simulink model "gyroscope"  (R2018a)
settings: Solver=VariableStepAuto  StartTime=0.0  StopTime=10.0  RelTol=1e-3
libraries: simulink_extras x3
settings Model: Creator=David  LastModifiedBy=David

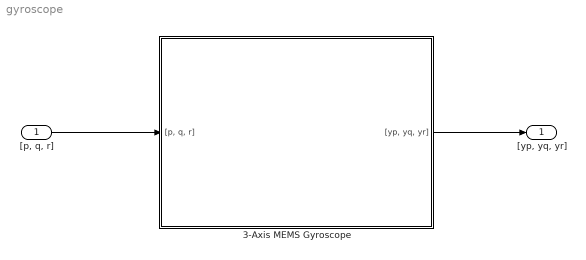
== system gyroscope ==
  "[p, q, r]" : Inport
  3-Axis MEMS Gyroscope : Subsystem  mask{SampleTime=0.01, gyroXNoiseDensity=0, gyroYNoiseDensity=0, gyroZNoiseDensity=0, gyroXBandwidthHz=1E06, gyroYBandwidthHz=1E06, gyroZBandwidthHz=1E06, gyroXInit=0, gyroYInit=0, gyroZInit=0, gyroXUpperSaturation=inf, gyroXLowerSaturation=-inf, gyroYUpperSaturation=inf, gyroYLowerSaturation=-inf, gyroZUpperSaturation=inf, gyroZLowerSaturation=-inf, gyroXResolution=1E-06, gyroYResolution=1E-06, gyroZResolution=1E-06}
      mask prompts: SampleTime "Gyroscope Sample Time (s)"; gyroXNoiseDensity "X Gyroscope Noise Density (rad/s/sqrt(Hz))"; gyroYNoiseDensity "Y Gyroscope Noise Density (rad/s/sqrt(Hz))"; gyroZNoiseDensity "Z Gyroscope Noise Density (rad/s/sqrt(Hz))"; gyroXBandwidthHz "X Gyroscope Bandwidth (Hz)"; gyroYBandwidthHz "Y Gyroscope Bandwidth (Hz)"; gyroZBandwidthHz "Z Gyroscope Bandwidth (Hz)"; gyroXInit "X Gyroscope Initial Condition (rad/s)"; gyroYInit "Y Gyroscope Initial Condition (rad/s)"; gyroZInit "Z Gyroscope Initial Condition (rad/s)"; gyroXUpperSaturation "X Gyroscope Measurement Upper Saturation Limit (rad/s)"; gyroXLowerSaturation "X Gyroscope Measurement Lower Saturation Limit (rad/s)"; gyroYUpperSaturation "Y Gyroscope Measurement Upper Saturation Limit (rad/s)"; gyroYLowerSaturation "Y Gyroscope Measurement Lower Saturation Limit (rad/s)"; gyroZUpperSaturation "Z Gyroscope Measurement Upper Saturation Limit (rad/s)"; gyroZLowerSaturation "Z Gyroscope Measurement Lower Saturation Limit (rad/s)"; gyroXResolution "X Gyroscope Resolution (rad/s)"; gyroYResolution "Y Gyroscope Resolution (rad/s)"; gyroZResolution "Z Gyroscope Resolution (rad/s)"
      mask DialogControl DescGroupVar Prompt: MEMS Gyroscope Model
      mask DialogControl DescTextVar Prompt: MEMS Gyroscope Model with White Noise Modelling
      mask DialogControl Container7 Prompt: System Characteristics
      mask DialogControl Container4 Prompt: Noise Characteristics
      mask DialogControl Container6 Prompt: Sensor Dynamics
      mask DialogControl Container9 Prompt: Bandwidth
      mask DialogControl Container10 Prompt: Initial Conditions
      mask DialogControl Container11 Prompt: Limits and Quantization
      mask DialogControl Container13 Prompt: Limits
      mask DialogControl Container14 Prompt: Quantization
      mask DialogControl Control3 Prompt: This can be calculated with the following equation:
      mask DialogControl Control2 Prompt: Physical Resolution = measurement_span/(2^resolution_bits - 1)
      mask Display:
      | image('mems_gyro.jpg')
      | 
      | color('red')
      | 
      | port_label('input', 1, '[p, q, r] (rad/s)', 'texMode', 'on')
      | 
      | port_label('output', 1, '[y_{gyro_p}, y_{gyro_q}, y_{gyro_r}] (rad/s)', 'texMode', 'on')
  "[yp, yq, yr]" : Outport
  wires:
  "[p, q, r]"/1 -> 3-Axis MEMS Gyroscope/1("[p, q, r]")
  3-Axis MEMS Gyroscope/1("[yp, yq, yr]") -> "[yp, yq, yr]"/1

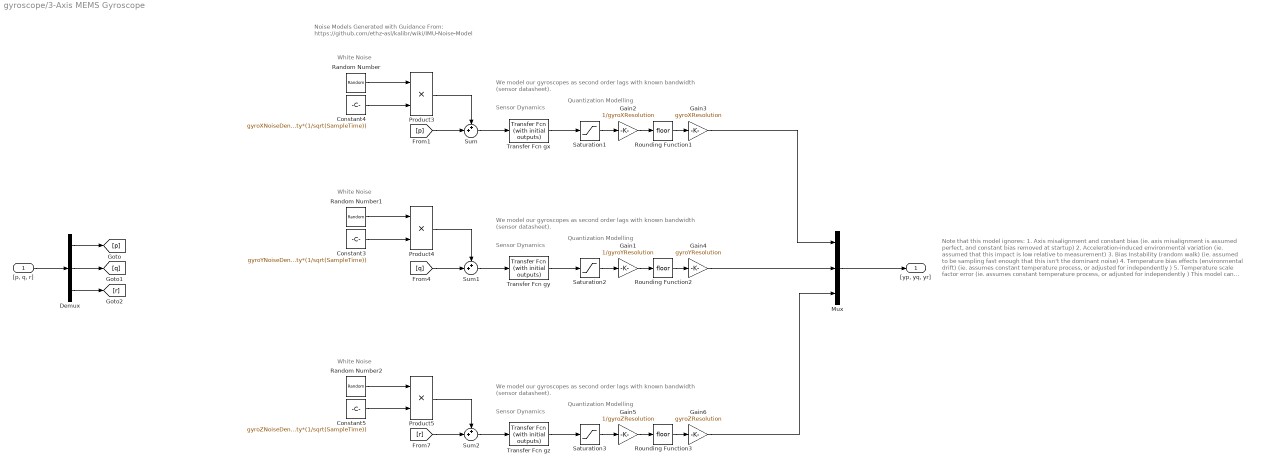
== system gyroscope/3-Axis MEMS Gyroscope ==
  note: White Noise
  note: Noise Models Generated with Guidance From:
      | https://github.com/ethz-asl/kalibr/wiki/IMU-Noise-Model
  note: White Noise
  note: White Noise
  note: We model our gyroscopes as second order lags with known bandwidth
      | (sensor datasheet).
  note: Quantization Modelling
  note: Sensor Dynamics
  note: Quantization Modelling
  note: Sensor Dynamics
  note: We model our gyroscopes as second order lags with known bandwidth
      | (sensor datasheet).
  note: Quantization Modelling
  note: We model our gyroscopes as second order lags with known bandwidth
      | (sensor datasheet).
  note: Sensor Dynamics
  note: Note that this model ignores:
      | 1. Axis misalignment and constant bias (ie. axis misalignment is assumed perfect, and constant bias removed at startup)
      | 2. Acceleration-induced environmental variation (ie. assumed that this impact is low relative to measurement)
      | 3. Bias Instability (random walk) (ie. assumed to be sampling fast enough that this isn't the dominant noise)
      | 4. Temperature bias effects (environmental drift) (ie. assumes constant temperature process, or adjusted for independently )
      | 5. Temperature scale factor error (ie. assumes constant temperature process, or adjusted for independently )
      |
      | This model can be extended by reviewing:
      | https://www.mathworks.com/help/fusion/ref/imusensor-system-object.html?searchHighlight=imuSensor&s_tid=doc_srchtitle
  "[p, q, r]" : Inport
  Constant3 : Constant  Value=gyroYNoiseDensity*(1/sqrt(SampleTime))
  Constant4 : Constant  Value=gyroXNoiseDensity*(1/sqrt(SampleTime))
  Constant5 : Constant  Value=gyroZNoiseDensity*(1/sqrt(SampleTime))
  Demux : Demux  Outputs=3
  Gain1 : Gain  Gain=1/gyroYResolution
  Gain2 : Gain  Gain=1/gyroXResolution
  Gain3 : Gain  Gain=gyroXResolution
  Gain4 : Gain  Gain=gyroYResolution
  Gain5 : Gain  Gain=1/gyroZResolution
  Gain6 : Gain  Gain=gyroZResolution
  Mux : Mux  Inputs=3
  Product3 : Product
  Product4 : Product
  Product5 : Product
  Random Number : RandomNumber  SampleTime=SampleTime
  Random Number1 : RandomNumber  SampleTime=SampleTime
  Random Number2 : RandomNumber  SampleTime=SampleTime
  Rounding Function1 : Rounding
  Rounding Function2 : Rounding
  Rounding Function3 : Rounding
  Saturation1 : Saturate  UpperLimit=gyroXUpperSaturation  LowerLimit=gyroXLowerSaturation
  Saturation2 : Saturate  UpperLimit=gyroYUpperSaturation  LowerLimit=gyroYLowerSaturation
  Saturation3 : Saturate  UpperLimit=gyroZUpperSaturation  LowerLimit=gyroZLowerSaturation
  Sum : Sum  Inputs=++|
  Sum1 : Sum  Inputs=++|
  Sum2 : Sum  Inputs=++|
  Transfer Fcn gx : simulink_extras/Additional Linear/Transfer Fcn (with initial outputs)  N=[(gyroXBandwidthHz*2*pi)^2]  D="[1,  2*gyroXBandwidthHz*2*pi, (gyroXBandwidthHz*2*pi)^2]"  Y0=gyroXInit  U0=gyroXInit
  Transfer Fcn gy : simulink_extras/Additional Linear/Transfer Fcn (with initial outputs)  N=[(gyroYBandwidthHz*2*pi)^2]  D="[1,  2*gyroYBandwidthHz*2*pi, (gyroYBandwidthHz*2*pi)^2]"  Y0=gyroYInit  U0=gyroYInit
  Transfer Fcn gz : simulink_extras/Additional Linear/Transfer Fcn (with initial outputs)  N=[(gyroZBandwidthHz*2*pi)^2]  D="[1,  2*gyroZBandwidthHz*2*pi, (gyroZBandwidthHz*2*pi)^2]"  Y0=gyroZInit  U0=gyroZInit
  "[yp, yq, yr]" : Outport
  wires:
  [p] -> Sum/2
  Demux/3 -> [r]
  Mux/1 -> "[yp, yq, yr]"/1
  [r] -> Sum2/2
  [q] -> Sum1/2
  Demux/1 -> [p]
  Demux/2 -> [q]
  "[p, q, r]"/1 -> Demux/1
  Random Number/1 -> Product3/1
  Product3/1 -> Sum/1
  Constant4/1 -> Product3/2
  Random Number1/1 -> Product4/1
  Constant3/1 -> Product4/2
  Product4/1 -> Sum1/1
  Product5/1 -> Sum2/1
  Constant5/1 -> Product5/2
  Random Number2/1 -> Product5/1
  Gain3/1 -> Mux/1
  Sum/1 -> Transfer Fcn gx/1
  Rounding Function1/1 -> Gain3/1
  Saturation1/1 -> Gain2/1
  Transfer Fcn gx/1 -> Saturation1/1
  Gain2/1 -> Rounding Function1/1
  Saturation2/1 -> Gain1/1
  Sum1/1 -> Transfer Fcn gy/1
  Gain4/1 -> Mux/2
  Rounding Function2/1 -> Gain4/1
  Gain1/1 -> Rounding Function2/1
  Transfer Fcn gy/1 -> Saturation2/1
  Sum2/1 -> Transfer Fcn gz/1
  Gain5/1 -> Rounding Function3/1
  Rounding Function3/1 -> Gain6/1
  Transfer Fcn gz/1 -> Saturation3/1
  Saturation3/1 -> Gain5/1
  Gain6/1 -> Mux/3
